simulink model "CSK_TS_PM_Message"  (R2014b)
settings: Solver=ode23s  StartTime=0.0  StopTime=801  RelTol=1e-12
values from neighbouring files (symbols this model uses):
  beta = 25.6    [RUN_021317.m]    (also in RUN_021417.m; RUN_022117.m)
  rho = 2    [RUN_021317.m]    (also in RUN_021417.m; RUN_022117.m)
  sig = 10    [RUN_021317.m]    (also in RUN_021417.m; RUN_022117.m)
  x0 = [.1,.2,.3]    [RUN_021317.m]    (also in RUN_021417.m; RUN_022117.m)
  z0 = x0    [RUN_021317.m]    (also in RUN_021417.m; RUN_022117.m)
libraries: simulink x3
settings Model: Creator=Dan  LastModifiedBy=Dan

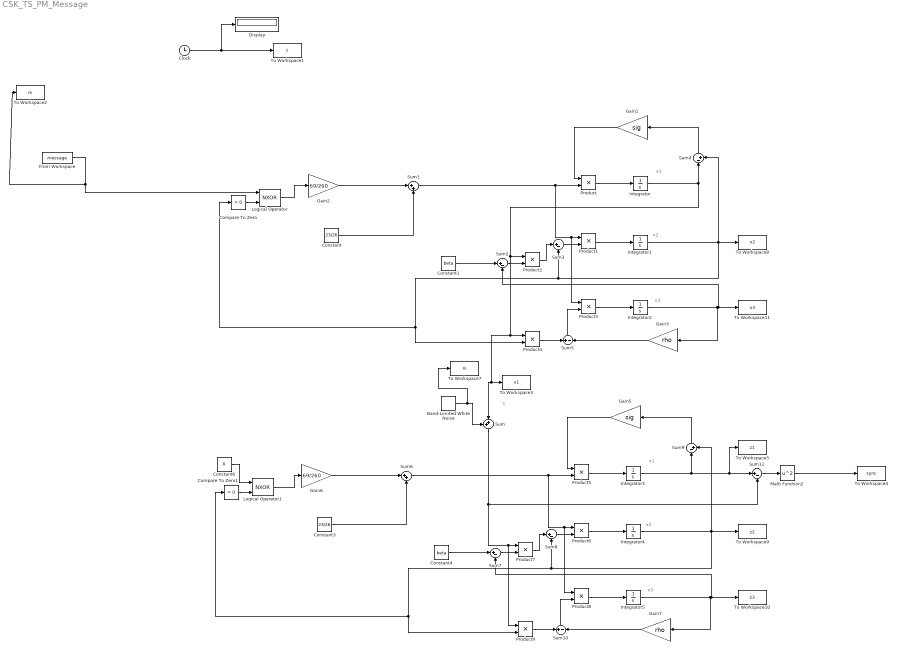
== system CSK_TS_PM_Message ==
  note: s
  note: x3
  note: x2
  note: x1
  note: x3
  note: x2
  note: x1
  Band-Limited White Noise : simulink/Sources/Band-Limited White Noise  Cov=NPower  Ts=0.1  seed=[23341]
  Clock : Clock
  Compare To Zero : simulink/Logic and Bit Operations/Compare To Zero  relop=<  OutDataTypeStr=boolean
  Compare To Zero1 : simulink/Logic and Bit Operations/Compare To Zero  relop=<  OutDataTypeStr=boolean
  Constant : Constant  Value=23/26
  Constant1 : Constant  Value=beta
  Constant3 : Constant  Value=23/26
  Constant4 : Constant  Value=beta
  Constant6 : Constant  Value=0
  Display : Display
      settings: Decimation=5
  From Workspace : FromWorkspace  VariableName=message  SampleTime=0  Interpolate=off  OutputAfterFinalValue=Holding final value
  Gain1 : Gain  Gain=sig
  Gain2 : Gain  Gain=69/260
  Gain3 : Gain  Gain=rho
  Gain5 : Gain  Gain=sig
  Gain6 : Gain  Gain=69/260
  Gain7 : Gain  Gain=rho
  Integrator : Integrator  InitialCondition=x0(1)
  Integrator1 : Integrator  InitialCondition=x0(2)
  Integrator2 : Integrator  InitialCondition=x0(3)
  Integrator3 : Integrator  InitialCondition=z0(1)
  Integrator4 : Integrator  InitialCondition=z0(2)
  Integrator5 : Integrator  InitialCondition=z0(3)
  Logical Operator : Logic  Operator=NXOR  AllPortsSameDT=off  OutDataTypeStr=boolean
  Logical Operator1 : Logic  Operator=NXOR  AllPortsSameDT=off  OutDataTypeStr=boolean
  Math Function2 : Math  Operator=square  SaturateOnIntegerOverflow=on
  Product{,1..9} (10 alike) : Product
  Sum : Sum  Inputs=++|
  Sum1 : Sum  Inputs=|++
  Sum10 : Sum  Inputs=+|-
  Sum{2..3,7..8,11} (5 alike) : Sum  Inputs=|+-
  Sum4 : Sum  Inputs=|-+
  Sum5 : Sum  Inputs=+|-
  Sum6 : Sum  Inputs=|++
  Sum9 : Sum  Inputs=|-+
  To Workspace1 : ToWorkspace  VariableName=t  SampleTime=-1
  To Workspace10 : ToWorkspace  VariableName=z3  SampleTime=-1
  To Workspace11 : ToWorkspace  VariableName=x3  SampleTime=-1
  To Workspace2 : ToWorkspace  VariableName=m  SampleTime=-1
  To Workspace3 : ToWorkspace  VariableName=x1  SampleTime=-1
  To Workspace4 : ToWorkspace  VariableName=sync  SampleTime=-1
  To Workspace5 : ToWorkspace  VariableName=z1  SampleTime=-1
  To Workspace7 : ToWorkspace  VariableName=ni  SampleTime=-1
  To Workspace8 : ToWorkspace  VariableName=x2  SampleTime=-1
  To Workspace9 : ToWorkspace  VariableName=z2  SampleTime=-1
  wires:
  Clock/1 -> Display/1, To Workspace1/1
  Sum4/1 -> Gain1/1
  Product/1 -> Integrator/1
  Gain1/1 -> Product/1
  From Workspace/1 -> To Workspace2/1, Logical Operator/1
  Constant/1 -> Sum1/2
  Sum1/1 -> Product3/1, Product1/1, Product/2
  Product2/1 -> Sum3/1
  Sum3/1 -> Product1/2
  Product1/1 -> Integrator1/1
  Sum2/1 -> Product2/2
  Constant1/1 -> Sum2/1
  Integrator2/1 -> To Workspace11/1, Sum2/2, Gain3/1
  Product3/1 -> Integrator2/1
  Integrator1/1 -> To Workspace8/1, Sum4/2, Sum3/2, Compare To Zero/1, Product4/2
  Compare To Zero/1 -> Logical Operator/2
  Logical Operator/1 -> Gain2/1
  Gain2/1 -> Sum1/1
  Gain3/1 -> Sum5/2
  Sum5/1 -> Product3/2
  Product4/1 -> Sum5/1
  Sum9/1 -> Gain5/1
  Product5/1 -> Integrator3/1
  Gain5/1 -> Product5/1
  Constant3/1 -> Sum6/2
  Sum6/1 -> Product8/1, Product6/1, Product5/2
  Product7/1 -> Sum8/1
  Sum8/1 -> Product6/2
  Product6/1 -> Integrator4/1
  Integrator3/1 -> To Workspace5/1, Sum11/1, Sum9/1
  Sum7/1 -> Product7/2
  Constant4/1 -> Sum7/1
  Integrator5/1 -> To Workspace10/1, Sum7/2, Gain7/1
  Product8/1 -> Integrator5/1
  Integrator4/1 -> Sum9/2, To Workspace9/1, Sum8/2, Compare To Zero1/1, Product9/2
  Logical Operator1/1 -> Gain6/1
  Gain6/1 -> Sum6/1
  Gain7/1 -> Sum10/2
  Sum10/1 -> Product8/2
  Product9/1 -> Sum10/1
  Constant6/1 -> Logical Operator1/1
  Integrator/1 -> Sum4/1, To Workspace3/1, Sum/2, Product4/1, Product2/1
  Sum11/1 -> Math Function2/1
  Math Function2/1 -> To Workspace4/1
  Band-Limited White Noise/1 -> To Workspace7/1, Sum/1
  Sum/1 -> Sum11/2, Product9/1, Product7/1
  Compare To Zero1/1 -> Logical Operator1/2
